simulink model "AttitudeDynamics"  (R2017b)
settings: Solver=VariableStepAuto  StartTime=0.0  StopTime=200  MaxStep=0.1  RelTol=1e-3  EnableMultiTasking=on
StopFcn:
  | attitudePlot = animateAttitude(rotmOut, 0.016);
  | attitudePlot.plotInit;
libraries: SatelliteLibrary x3
settings Model: Creator=Huib  LastModifiedBy=Huib
settings DataIOCC: LimitDataPoints=on
settings OptimizationCC: LifeSpan=inf
settings DebuggingCC: AllowSymbolicDim=off  SFUnexpectedBacktrackingDiag=warning  SFNoUnconditionalDefaultTransitionDiag=warning  SFExecutionAtInitializationDiag=none
settings ModelReferenceCC: PropagateSignalLabelsOutOfModel=off
settings CodeAppCC: StateflowObjectComments=on
settings GRTTargetCC: TargetLangStandard=C89/C90 (ANSI)
settings ConfigComp: CovMetricSettings=dw  CovHtmlReporting=on  CovSaveCumulativeToWorkspaceVar=on  CovSaveSingleToWorkspaceVar=on  CovExternalEMLEnable=off

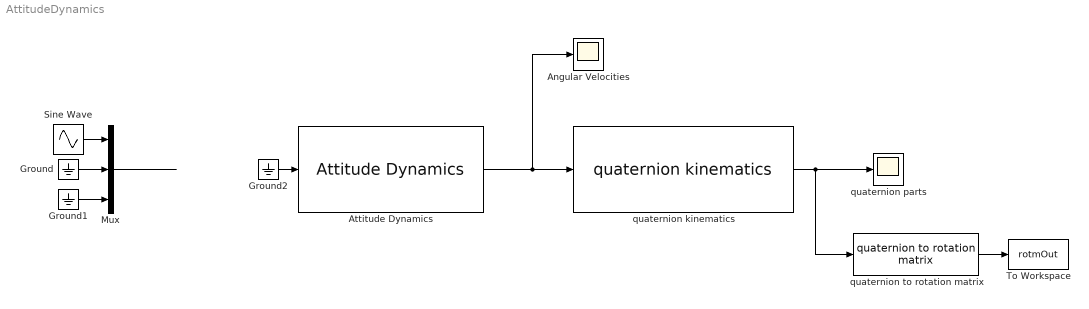
== system AttitudeDynamics ==
  Angular Velocities : Scope
  Attitude Dynamics : SatelliteLibrary/Attitude Dynamics  J11=1.5  J22=1  J33=0.5  omega0=[0.0 3 0.05]
  Ground : Ground
  Ground1 : Ground
  Ground2 : Ground
  Mux : Mux  Inputs=3
  Sine Wave : Sin  Amplitude=0.5  Frequency=2  SampleTime=0
  To Workspace : ToWorkspace  VariableName=rotmOut  SaveFormat=Timeseries  SampleTime=-1
  quaternion kinematics : SatelliteLibrary/quaternion kinematics  q_0=[0 0 0 1]
  quaternion parts : Scope
  quaternion to rotation matrix : SatelliteLibrary/quaternion to rotation matrix
      settings: SourceProductName=Stateflow  SourceProductBaseCode=SF
  wires:
  Mux/1 -> ?
  Attitude Dynamics/1 -> quaternion kinematics/1, Angular Velocities/1
  quaternion kinematics/1 -> quaternion to rotation matrix/1, quaternion parts/1
  quaternion to rotation matrix/1 -> To Workspace/1
  Sine Wave/1 -> Mux/1
  Ground/1 -> Mux/2
  Ground1/1 -> Mux/3
  Ground2/1 -> Attitude Dynamics/1
